simulink model "Test_Memory_Block_Word"  (R2023a)
settings: Solver=ode45  StartTime=0.0  StopTime=len  RelTol=1e-3  EnableMultiTasking=on
libraries: Miscellaneous x2, Memory_Blocks_Lib x1
settings Model: Creator=N  LastModifiedBy=Jozko Mrkvicka
settings SolverCC: AlgebraicLoopSolver=TrustRegion
settings DataIOCC: SaveFormat=Array  ReturnWorkspaceOutputs=off
settings OptimizationCC: LifeSpan=inf
settings DebuggingCC: UnconnectedInputMsg=warning  UnconnectedOutputMsg=warning  UnconnectedLineMsg=warning  SFUnexpectedBacktrackingDiag=warning  SFNoUnconditionalDefaultTransitionDiag=warning  ArithmeticOperatorsInVariantConditions=warning
settings HardwareCC: ProdWordSize=32
settings ModelReferenceCC: EnableRefExpFcnMdlSchedulingChecks=on
settings SFSimCC: SimUseLocalCustomCode=off  CustomCodeUndefinedFunction=UseInterfaceOnly
settings RTWCC: RTWUseLocalCustomCode=off
settings CodeAppCC: StateflowObjectComments=on
settings GRTTargetCC: TargetLangStandard=C89/C90 (ANSI)
settings ConfigComp: CovMetricSettings=dw  CovSaveCumulativeToWorkspaceVar=on  CovSaveSingleToWorkspaceVar=on  CovExternalEMLEnable=off

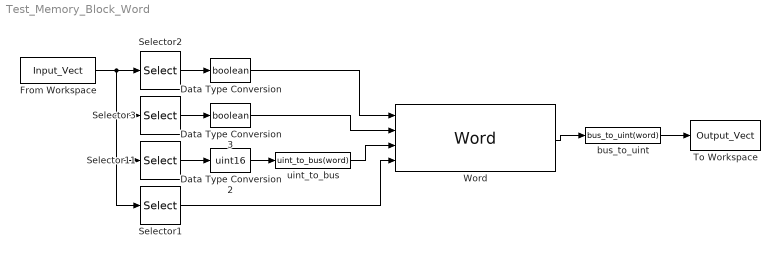
== system Test_Memory_Block_Word ==
  Data Type Conversion : DataTypeConversion  OutDataTypeStr=boolean  SaturateOnIntegerOverflow=off  RndMeth=Floor
  Data Type Conversion2 : DataTypeConversion  OutDataTypeStr=uint16  SaturateOnIntegerOverflow=off  RndMeth=Floor
  Data Type Conversion3 : DataTypeConversion  OutDataTypeStr=boolean  SaturateOnIntegerOverflow=off  RndMeth=Floor
  From Workspace : FromWorkspace  VariableName=Input_Vect  SampleTime=1  Interpolate=off  ZeroCross=off  OutputAfterFinalValue=Holding final value
  Selector1 : Selector  IndexMode=Zero-based  InputPortWidth=4  IndexOptions=Index vector (dialog)  Indices=3  OutputSizes=1
  Selector11 : Selector  IndexMode=Zero-based  InputPortWidth=4  IndexOptions=Index vector (dialog)  Indices=2  OutputSizes=1
  Selector2 : Selector  IndexMode=Zero-based  InputPortWidth=4  IndexOptions=Index vector (dialog)  Indices=0  OutputSizes=1
  Selector3 : Selector  IndexMode=Zero-based  InputPortWidth=4  IndexOptions=Index vector (dialog)  Indices=1  OutputSizes=1
  To Workspace : ToWorkspace  VariableName=Output_Vect  SampleTime=1
  Word : Memory_Blocks_Lib/Word  SystemSampleTime=-1  VariantActivationTime=update diagram  Latency=0  AutoFrameSizeCalculation=off
  bus_to_uint : Miscellaneous/bus_to_uint(word)
  uint_to_bus : Miscellaneous/uint_to_bus(word)
  wires:
  Word/1 -> bus_to_uint/1
  bus_to_uint/1 -> To Workspace/1
  Selector11/1 -> Data Type Conversion2/1
  Selector2/1 -> Data Type Conversion/1
  Selector1/1 -> Word/4
  From Workspace/1 -> Selector3/1, Selector1/1, Selector11/1, Selector2/1
  Data Type Conversion/1 -> Word/1
  Data Type Conversion2/1 -> uint_to_bus/1
  Selector3/1 -> Data Type Conversion3/1
  Data Type Conversion3/1 -> Word/2
  uint_to_bus/1 -> Word/3
